simulink model "TwoLoopANNC_Integral_Paper"  (R2020b)
settings: Solver=ode4  StartTime=0.0  StopTime=100  FixedStep=1e-3  RelTol=1e-3
settings Model: Creator=Ivan Lopez  LastModifiedBy=Ivan Lopez

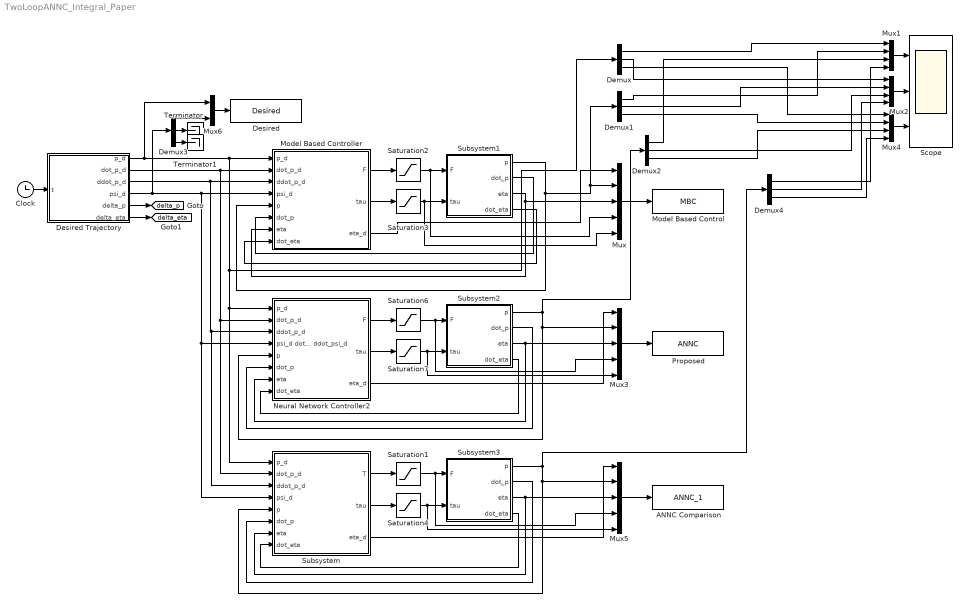
== system TwoLoopANNC_Integral_Paper ==
  ANNC Comparison : ToWorkspace  VariableName=ANNC_1  SaveFormat=Structure With Time  SampleTime=-1
  Clock : Clock
  Demux{,1..4} (5 alike) : Demux  Outputs=3
  Desired : ToWorkspace  VariableName=Desired  SaveFormat=Structure With Time  SampleTime=-1
  Desired Trajectory : MATLAB Function  TreatAsAtomicUnit=on
  Model Based Control : ToWorkspace  VariableName=MBC  SaveFormat=Structure With Time  SampleTime=-1
  Model Based Controller : Subsystem
  Mux : Mux  Inputs=5
  Mux1 : Mux
  Mux2 : Mux
  Mux3 : Mux  Inputs=5
  Mux4 : Mux
  Mux5 : Mux  Inputs=5
  Mux6 : Mux  Inputs=2
  Neural Network Controller2 : Subsystem
  Proposed : ToWorkspace  VariableName=ANNC  SaveFormat=Structure With Time  SampleTime=-1
  Saturation1 : Saturate  UpperLimit=34.4  LowerLimit=0
  Saturation2 : Saturate  UpperLimit=34.4  LowerLimit=0
  Saturation3 : Saturate  UpperLimit=1.72  LowerLimit=-1.72
  Saturation4 : Saturate  UpperLimit=1.72  LowerLimit=-1.72
  Saturation6 : Saturate  UpperLimit=34.4  LowerLimit=0
  Saturation7 : Saturate  UpperLimit=1.72  LowerLimit=-1.72
  Scope : Scope  NumInputPorts=3
  Subsystem : Subsystem
  Subsystem1 : Subsystem
  Subsystem2 : Subsystem
  Subsystem3 : Subsystem
  Terminator : Terminator
  Terminator1 : Terminator
  tag scope: delta_eta=global, delta_p=global
  wires:
  Neural Network Controller2/3(eta_d) -> Mux3/1
  Subsystem2/2(dot_p) -> Neural Network Controller2/6(dot_p)
  Subsystem2/4(dot_eta) -> Neural Network Controller2/8(dot_eta)
  Saturation3/1 -> Mux/5, Subsystem1/2(tau)
  Neural Network Controller2/2(tau) -> Saturation7/1
  Subsystem2/3(eta) -> Mux3/3, Neural Network Controller2/7(eta)
  Saturation7/1 -> Subsystem2/2(tau), Mux3/5
  Mux3/1 -> Proposed/1
  Subsystem1/1(p) -> Model Based Controller/5(p), Demux1/1, Mux/2
  Model Based Controller/3(eta_d) -> Mux/1
  Subsystem1/3(eta) -> Mux/3, Model Based Controller/7(eta)
  Model Based Controller/1(F) -> Saturation2/1
  Clock/1 -> Desired Trajectory/1(t)
  Saturation2/1 -> Mux/4, Subsystem1/1(F)
  Neural Network Controller2/1(F) -> Saturation6/1
  Desired Trajectory/3(ddot_p_d) -> Subsystem/3(ddot_p_d), Neural Network Controller2/3(ddot_p_d), Model Based Controller/3(ddot_p_d)
  Desired Trajectory/2(dot_p_d) -> Subsystem/2(dot_p_d), Neural Network Controller2/2(dot_p_d), Model Based Controller/2(dot_p_d)
  Mux/1 -> Model Based Control/1
  Saturation6/1 -> Subsystem2/1(F), Mux3/4
  Subsystem1/2(dot_p) -> Model Based Controller/6(dot_p)
  Desired Trajectory/1(p_d) -> Subsystem/1(p_d), Neural Network Controller2/1(p_d), Demux/1, Model Based Controller/1(p_d), Mux6/1
  Model Based Controller/2(tau) -> Saturation3/1
  Desired Trajectory/4(psi_d) -> Subsystem/4(psi_d), Neural Network Controller2/4(psi_d dot_psi_d ddot_psi_d), Model Based Controller/4(psi_d), Demux3/1
  Desired Trajectory/5(delta_p) -> [delta_p]
  Desired Trajectory/6(delta_eta) -> [delta_eta]
  Subsystem1/4(dot_eta) -> Model Based Controller/8(dot_eta)
  Mux1/1 -> Scope/1
  Mux2/1 -> Scope/2
  Mux4/1 -> Scope/3
  Demux/1 -> Mux1/1
  Demux1/1 -> Mux1/2
  Demux/2 -> Mux2/1
  Demux1/2 -> Mux2/2
  Demux/3 -> Mux4/1
  Demux1/3 -> Mux4/2
  Subsystem2/1(p) -> Demux2/1, Mux3/2, Neural Network Controller2/5(p)
  Demux2/1 -> Mux1/3
  Demux2/2 -> Mux2/3
  Demux2/3 -> Mux4/3
  Subsystem/3(eta_d) -> Mux5/1
  Subsystem3/1(p) -> Demux4/1, Subsystem/5(p), Mux5/2
  Saturation1/1 -> Subsystem3/1(F), Mux5/4
  Subsystem/1(T) -> Saturation1/1
  Subsystem3/4(dot_eta) -> Subsystem/8(dot_eta)
  Subsystem3/3(eta) -> Subsystem/7(eta), Mux5/3
  Mux5/1 -> ANNC Comparison/1
  Saturation4/1 -> Subsystem3/2(tau), Mux5/5
  Subsystem3/2(dot_p) -> Subsystem/6(dot_p)
  Subsystem/2(tau) -> Saturation4/1
  Mux6/1 -> Desired/1
  Demux3/1 -> Mux6/2
  Demux3/2 -> Terminator/1
  Demux3/3 -> Terminator1/1
  Demux4/1 -> Mux1/4
  Demux4/2 -> Mux2/4
  Demux4/3 -> Mux4/4

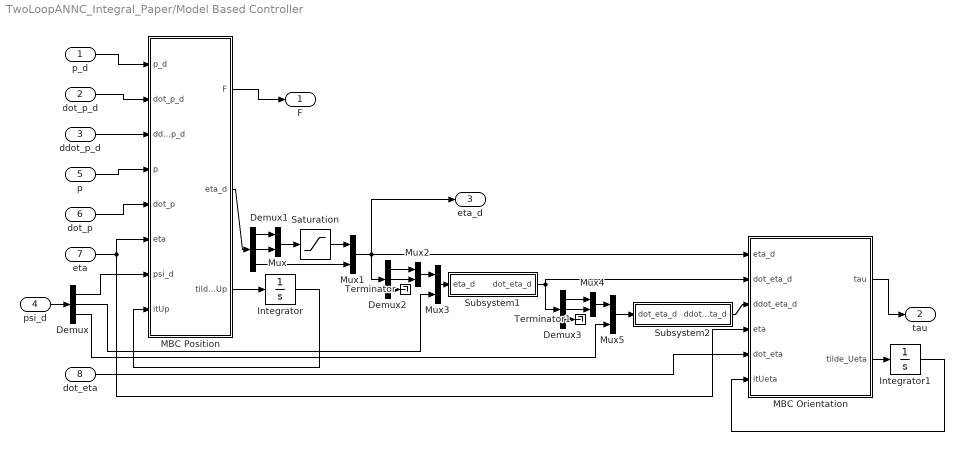
== system TwoLoopANNC_Integral_Paper/Model Based Controller ==
  p_d : Inport
  dot_p_d : Inport  Port=2
  ddot_p_d : Inport  Port=3
  psi_d : Inport  Port=4
  p : Inport  Port=5
  dot_p : Inport  Port=6
  eta : Inport  Port=7
  dot_eta : Inport  Port=8
  Demux{,1..3} (4 alike) : Demux  Outputs=3
  Integrator : Integrator  InitialCondition=[0;0;0]
  Integrator1 : Integrator  InitialCondition=[0;0;0]
  MBC Orientation : MATLAB Function  TreatAsAtomicUnit=on
  MBC Position : MATLAB Function  TreatAsAtomicUnit=on
  Mux{,1..5} (6 alike) : Mux  Inputs=2
  Saturation : Saturate  UpperLimit=20*pi/180  LowerLimit=-20*pi/180
  Subsystem1 : Subsystem
  Subsystem2 : Subsystem
  Terminator : Terminator
  Terminator1 : Terminator
  F : Outport
  tau : Outport  Port=2
  eta_d : Outport  Port=3
  wires:
  psi_d/1 -> Demux/1
  Subsystem1/1(dot_eta_d) -> Demux3/1, MBC Orientation/2(dot_eta_d)
  Subsystem2/1(ddot_eta_d) -> MBC Orientation/3(ddot_eta_d)
  MBC Position/1(F) -> F/1
  eta/1 -> MBC Orientation/4(eta), MBC Position/6(eta)
  ddot_p_d/1 -> MBC Position/3(ddot_p_d)
  MBC Orientation/1(tau) -> tau/1
  p/1 -> MBC Position/4(p)
  dot_p/1 -> MBC Position/5(dot_p)
  p_d/1 -> MBC Position/1(p_d)
  dot_eta/1 -> MBC Orientation/5(dot_eta)
  dot_p_d/1 -> MBC Position/2(dot_p_d)
  Mux1/1 -> Demux2/1, eta_d/1, MBC Orientation/1(eta_d)
  Demux/1 -> MBC Position/7(psi_d)
  MBC Position/2(eta_d) -> Demux1/1
  Demux1/2 -> Mux/2
  Demux1/1 -> Mux/1
  Mux/1 -> Saturation/1
  Saturation/1 -> Mux1/1
  Demux1/3 -> Mux1/2
  Demux2/2 -> Mux2/2
  Demux2/1 -> Mux2/1
  Mux2/1 -> Mux3/1
  Mux3/1 -> Subsystem1/1(eta_d)
  Demux/2 -> Mux3/2
  Demux2/3 -> Terminator/1
  Demux3/2 -> Mux4/2
  Mux5/1 -> Subsystem2/1(dot_eta_d)
  Mux4/1 -> Mux5/1
  Demux3/1 -> Mux4/1
  Demux3/3 -> Terminator1/1
  Demux/3 -> Mux5/2
  MBC Position/3(tilde_Up) -> Integrator/1
  Integrator/1 -> MBC Position/8(itUp)
  MBC Orientation/2(tilde_Ueta) -> Integrator1/1
  Integrator1/1 -> MBC Orientation/6(itUeta)

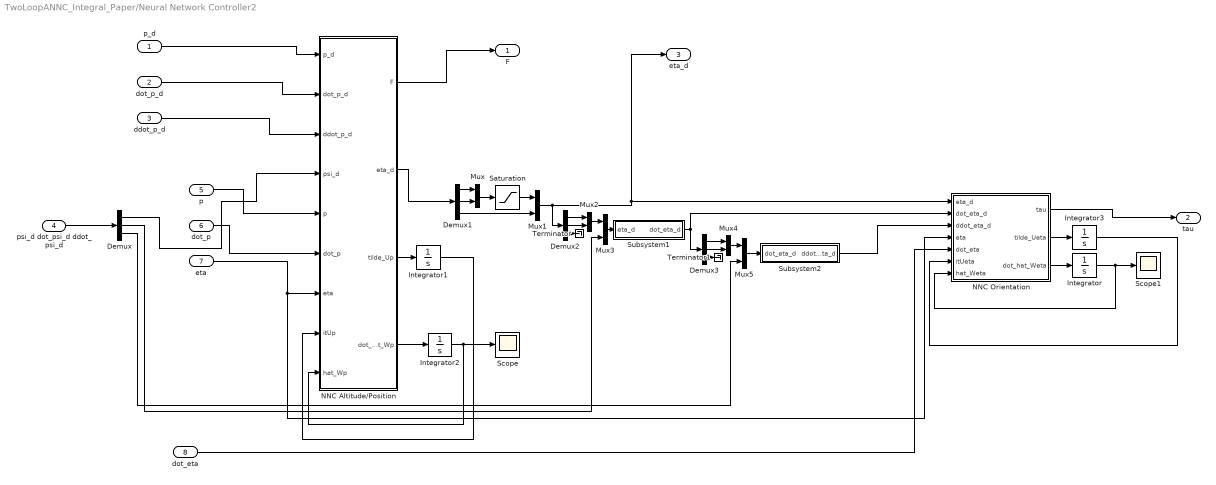
== system TwoLoopANNC_Integral_Paper/Neural Network Controller2 ==
  p_d : Inport
  dot_p_d : Inport  Port=2
  ddot_p_d : Inport  Port=3
  psi_d dot_psi_d ddot_psi_d : Inport  Port=4
  p : Inport  Port=5
  dot_p : Inport  Port=6
  eta : Inport  Port=7
  dot_eta : Inport  Port=8
  Demux{,1..3} (4 alike) : Demux  Outputs=3
  Integrator : Integrator  InitialCondition=zeros(10,3)
  Integrator1 : Integrator  InitialCondition=[0;0;0]
  Integrator2 : Integrator  InitialCondition=zeros(10,3)
  Integrator3 : Integrator  InitialCondition=[0;0;0]
  Mux{,1..5} (6 alike) : Mux  Inputs=2
  NNC Altitude/Position : MATLAB Function  TreatAsAtomicUnit=on
  NNC Orientation : MATLAB Function  TreatAsAtomicUnit=on
  Saturation : Saturate  UpperLimit=20*pi/180  LowerLimit=-20*pi/180
  Scope : Scope
  Scope1 : Scope
  Subsystem1 : Subsystem
  Subsystem2 : Subsystem
  Terminator : Terminator
  Terminator1 : Terminator
  F : Outport
  tau : Outport  Port=2
  eta_d : Outport  Port=3
  wires:
  NNC Altitude/Position/4(dot_hat_Wp) -> Integrator2/1
  Integrator/1 -> Scope1/1, NNC Orientation/7(hat_Weta)
  NNC Orientation/3(dot_hat_Weta) -> Integrator/1
  Integrator2/1 -> Scope/1, NNC Altitude/Position/9(hat_Wp)
  psi_d dot_psi_d ddot_psi_d/1 -> Demux/1
  Demux3/3 -> Terminator1/1
  Mux4/1 -> Mux5/1
  Demux3/1 -> Mux4/1
  Demux3/2 -> Mux4/2
  Demux/3 -> Mux5/2
  Demux/2 -> Mux3/2
  NNC Altitude/Position/2(eta_d) -> Demux1/1
  Demux1/1 -> Mux/1
  Demux2/2 -> Mux2/2
  Mux3/1 -> Subsystem1/1(eta_d)
  Demux1/3 -> Mux1/2
  Mux2/1 -> Mux3/1
  Demux2/3 -> Terminator/1
  Saturation/1 -> Mux1/1
  Demux1/2 -> Mux/2
  Mux5/1 -> Subsystem2/1(dot_eta_d)
  Demux2/1 -> Mux2/1
  Subsystem1/1(dot_eta_d) -> NNC Orientation/2(dot_eta_d), Demux3/1
  Mux1/1 -> NNC Orientation/1(eta_d), eta_d/1, Demux2/1
  Mux/1 -> Saturation/1
  Subsystem2/1(ddot_eta_d) -> NNC Orientation/3(ddot_eta_d)
  Demux/1 -> NNC Altitude/Position/4(psi_d)
  NNC Orientation/1(tau) -> tau/1
  NNC Altitude/Position/1(F) -> F/1
  dot_p_d/1 -> NNC Altitude/Position/2(dot_p_d)
  p_d/1 -> NNC Altitude/Position/1(p_d)
  eta/1 -> NNC Orientation/4(eta), NNC Altitude/Position/7(eta)
  p/1 -> NNC Altitude/Position/5(p)
  dot_p/1 -> NNC Altitude/Position/6(dot_p)
  dot_eta/1 -> NNC Orientation/5(dot_eta)
  ddot_p_d/1 -> NNC Altitude/Position/3(ddot_p_d)
  NNC Altitude/Position/3(tilde_Up) -> Integrator1/1
  Integrator1/1 -> NNC Altitude/Position/8(itUp)
  NNC Orientation/2(tilde_Ueta) -> Integrator3/1
  Integrator3/1 -> NNC Orientation/6(itUeta)

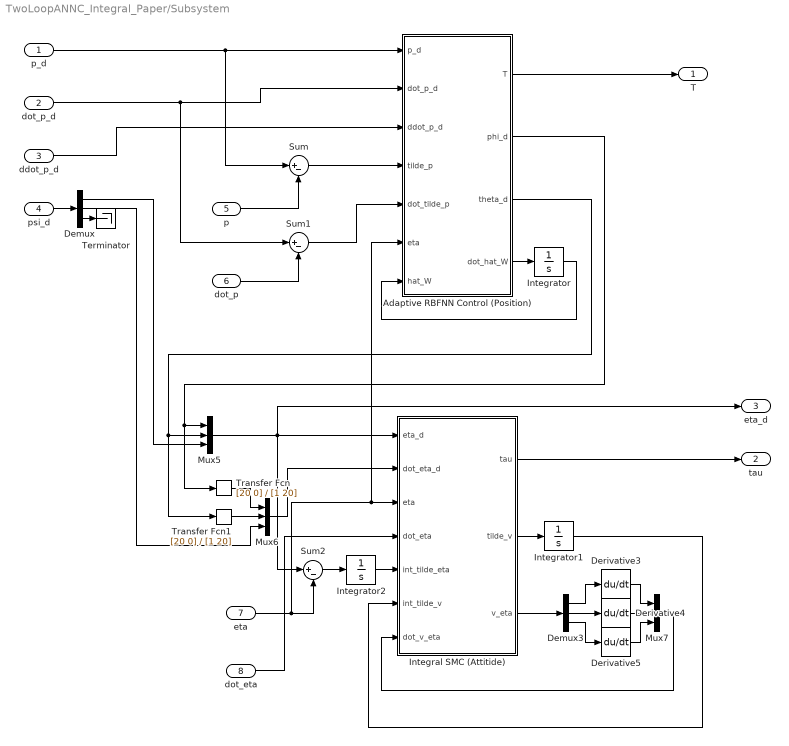
== system TwoLoopANNC_Integral_Paper/Subsystem ==
  p_d : Inport
  dot_p_d : Inport  Port=2
  ddot_p_d : Inport  Port=3
  psi_d : Inport  Port=4
  p : Inport  Port=5
  dot_p : Inport  Port=6
  eta : Inport  Port=7
  dot_eta : Inport  Port=8
  Adaptive RBFNN Control (Position) : MATLAB Function  TreatAsAtomicUnit=on
  Demux : Demux  Outputs=3
  Demux3 : Demux  Outputs=3
  Derivative3 : Derivative
  Derivative4 : Derivative
  Derivative5 : Derivative
  Integral SMC (Attitide) : MATLAB Function  TreatAsAtomicUnit=on
  Integrator : Integrator  InitialCondition=0.005*ones(7,3)
  Integrator1 : Integrator  InitialCondition=[0;0;0]
  Integrator2 : Integrator  InitialCondition=[0;0;0]
  Mux5 : Mux  Inputs=3
  Mux6 : Mux  Inputs=3
  Mux7 : Mux  Inputs=3
  Sum : Sum  Inputs=|+-
  Sum1 : Sum  Inputs=|+-
  Sum2 : Sum  Inputs=|+-
  Terminator : Terminator
  Transfer Fcn : TransferFcn  Numerator=[20 0]  Denominator=[1 20]
  Transfer Fcn1 : TransferFcn  Numerator=[20 0]  Denominator=[1 20]
  T : Outport
  tau : Outport  Port=2
  eta_d : Outport  Port=3
  wires:
  Demux3/1 -> Derivative3/1
  Adaptive RBFNN Control (Position)/3(theta_d) -> Transfer Fcn1/1, Mux5/2
  Integral SMC (Attitide)/1(tau) -> tau/1
  Demux/1 -> Mux5/3
  Adaptive RBFNN Control (Position)/2(phi_d) -> Transfer Fcn/1, Mux5/1
  eta/1 -> Adaptive RBFNN Control (Position)/6(eta), Integral SMC (Attitide)/3(eta), Sum2/2
  Mux7/1 -> Integral SMC (Attitide)/7(dot_v_eta)
  Demux3/3 -> Derivative5/1
  Sum1/1 -> Adaptive RBFNN Control (Position)/5(dot_tilde_p)
  Integral SMC (Attitide)/2(tilde_v) -> Integrator1/1
  Integrator1/1 -> Integral SMC (Attitide)/6(int_tilde_v)
  Derivative5/1 -> Mux7/3
  Mux5/1 -> eta_d/1, Sum2/1, Integral SMC (Attitide)/1(eta_d)
  Adaptive RBFNN Control (Position)/4(dot_hat_W) -> Integrator/1
  Transfer Fcn/1 -> Mux6/1
  Integral SMC (Attitide)/3(v_eta) -> Demux3/1
  Demux3/2 -> Derivative4/1
  dot_p_d/1 -> Sum1/1, Adaptive RBFNN Control (Position)/2(dot_p_d)
  Sum2/1 -> Integrator2/1
  Integrator/1 -> Adaptive RBFNN Control (Position)/7(hat_W)
  Derivative3/1 -> Mux7/1
  Derivative4/1 -> Mux7/2
  p/1 -> Sum/2
  dot_eta/1 -> Integral SMC (Attitide)/4(dot_eta)
  Transfer Fcn1/1 -> Mux6/2
  dot_p/1 -> Sum1/2
  Sum/1 -> Adaptive RBFNN Control (Position)/4(tilde_p)
  Mux6/1 -> Integral SMC (Attitide)/2(dot_eta_d)
  Integrator2/1 -> Integral SMC (Attitide)/5(int_tilde_eta)
  p_d/1 -> Sum/1, Adaptive RBFNN Control (Position)/1(p_d)
  ddot_p_d/1 -> Adaptive RBFNN Control (Position)/3(ddot_p_d)
  Adaptive RBFNN Control (Position)/1(T) -> T/1
  psi_d/1 -> Demux/1
  Demux/2 -> Mux6/3
  Demux/3 -> Terminator/1

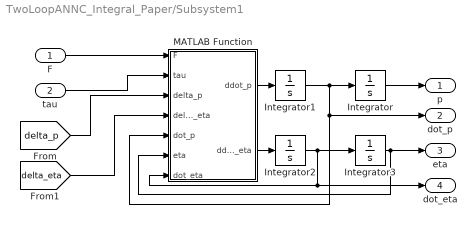
== system TwoLoopANNC_Integral_Paper/Subsystem1 ==
  F : Inport
  tau : Inport  Port=2
  Integrator : Integrator  InitialCondition=[0;0;0.3]  LimitOutput=on  UpperSaturationLimit=[inf;inf;inf]  LowerSaturationLimit=[-inf;-inf;0.3]
  Integrator1 : Integrator  InitialCondition=[0;0;0]
  Integrator2 : Integrator  InitialCondition=[0;0;0]
  Integrator3 : Integrator  InitialCondition=[0;0;0]  LimitOutput=on  UpperSaturationLimit=[pi/2; pi/2; inf]  LowerSaturationLimit=[-pi/2; -pi/2; -inf]
  MATLAB Function : MATLAB Function  TreatAsAtomicUnit=on
  p : Outport
  dot_p : Outport  Port=2
  eta : Outport  Port=3
  dot_eta : Outport  Port=4
  wires:
  [delta_p] -> MATLAB Function/3(delta_p)
  [delta_eta] -> MATLAB Function/4(delta_eta)
  F/1 -> MATLAB Function/1(F)
  Integrator3/1 -> MATLAB Function/6(eta), eta/1
  Integrator1/1 -> dot_p/1, MATLAB Function/5(dot_p), Integrator/1
  MATLAB Function/2(ddot_eta) -> Integrator2/1
  MATLAB Function/1(ddot_p) -> Integrator1/1
  tau/1 -> MATLAB Function/2(tau)
  Integrator2/1 -> Integrator3/1, dot_eta/1, MATLAB Function/7(dot_eta)
  Integrator/1 -> p/1

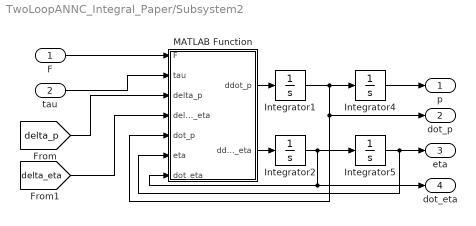
== system TwoLoopANNC_Integral_Paper/Subsystem2 ==
  F : Inport
  tau : Inport  Port=2
  Integrator1 : Integrator  InitialCondition=[0;0;0]
  Integrator2 : Integrator  InitialCondition=[0;0;0]
  Integrator4 : Integrator  InitialCondition=[0;0;0.3]  LimitOutput=on  UpperSaturationLimit=[inf;inf;inf]  LowerSaturationLimit=[-inf;-inf;0.3]
  Integrator5 : Integrator  InitialCondition=[0;0;0]  LimitOutput=on  UpperSaturationLimit=[pi/2; pi/2; inf]  LowerSaturationLimit=[-pi/2; -pi/2; -inf]
  MATLAB Function : MATLAB Function  TreatAsAtomicUnit=on
  p : Outport
  dot_p : Outport  Port=2
  eta : Outport  Port=3
  dot_eta : Outport  Port=4
  wires:
  [delta_p] -> MATLAB Function/3(delta_p)
  [delta_eta] -> MATLAB Function/4(delta_eta)
  F/1 -> MATLAB Function/1(F)
  MATLAB Function/2(ddot_eta) -> Integrator2/1
  MATLAB Function/1(ddot_p) -> Integrator1/1
  tau/1 -> MATLAB Function/2(tau)
  Integrator4/1 -> p/1
  Integrator5/1 -> eta/1, MATLAB Function/6(eta)
  Integrator1/1 -> Integrator4/1, dot_p/1, MATLAB Function/5(dot_p)
  Integrator2/1 -> Integrator5/1, dot_eta/1, MATLAB Function/7(dot_eta)

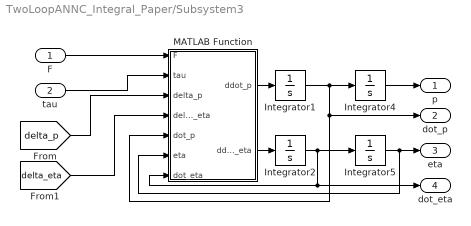
== system TwoLoopANNC_Integral_Paper/Subsystem3 ==
  F : Inport
  tau : Inport  Port=2
  Integrator1 : Integrator  InitialCondition=[0;0;0]
  Integrator2 : Integrator  InitialCondition=[0;0;0]
  Integrator4 : Integrator  InitialCondition=[0;0;0.3]  LimitOutput=on  UpperSaturationLimit=[inf;inf;inf]  LowerSaturationLimit=[-inf;-inf;0.3]
  Integrator5 : Integrator  InitialCondition=[0;0;0]  LimitOutput=on  UpperSaturationLimit=[pi/2; pi/2; inf]  LowerSaturationLimit=[-pi/2; -pi/2; -inf]
  MATLAB Function : MATLAB Function  TreatAsAtomicUnit=on
  p : Outport
  dot_p : Outport  Port=2
  eta : Outport  Port=3
  dot_eta : Outport  Port=4
  wires:
  [delta_p] -> MATLAB Function/3(delta_p)
  [delta_eta] -> MATLAB Function/4(delta_eta)
  F/1 -> MATLAB Function/1(F)
  MATLAB Function/2(ddot_eta) -> Integrator2/1
  MATLAB Function/1(ddot_p) -> Integrator1/1
  tau/1 -> MATLAB Function/2(tau)
  Integrator4/1 -> p/1
  Integrator5/1 -> eta/1, MATLAB Function/6(eta)
  Integrator1/1 -> Integrator4/1, dot_p/1, MATLAB Function/5(dot_p)
  Integrator2/1 -> Integrator5/1, dot_eta/1, MATLAB Function/7(dot_eta)

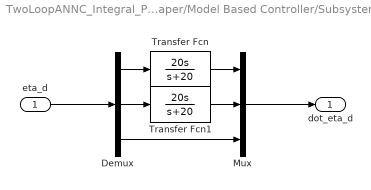
== system TwoLoopANNC_Integral_Paper/Model Based Controller/Subsystem1 ==
  eta_d : Inport
  Demux : Demux  Outputs=3
  Mux : Mux  Inputs=3
  Transfer Fcn : TransferFcn  Numerator=[20 0]  Denominator=[1 20]
  Transfer Fcn1 : TransferFcn  Numerator=[20 0]  Denominator=[1 20]
  dot_eta_d : Outport
  wires:
  Demux/2 -> Transfer Fcn1/1
  Demux/3 -> Mux/3
  Demux/1 -> Transfer Fcn/1
  Transfer Fcn/1 -> Mux/1
  Transfer Fcn1/1 -> Mux/2
  Mux/1 -> dot_eta_d/1
  eta_d/1 -> Demux/1

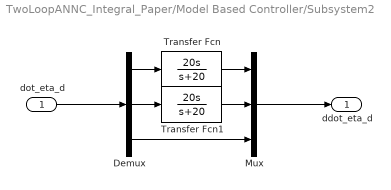
== system TwoLoopANNC_Integral_Paper/Model Based Controller/Subsystem2 ==
  dot_eta_d : Inport
  Demux : Demux  Outputs=3
  Mux : Mux  Inputs=3
  Transfer Fcn : TransferFcn  Numerator=[20 0]  Denominator=[1 20]
  Transfer Fcn1 : TransferFcn  Numerator=[20 0]  Denominator=[1 20]
  ddot_eta_d : Outport
  wires:
  Demux/3 -> Mux/3
  Transfer Fcn1/1 -> Mux/2
  Demux/2 -> Transfer Fcn1/1
  Demux/1 -> Transfer Fcn/1
  Transfer Fcn/1 -> Mux/1
  dot_eta_d/1 -> Demux/1
  Mux/1 -> ddot_eta_d/1

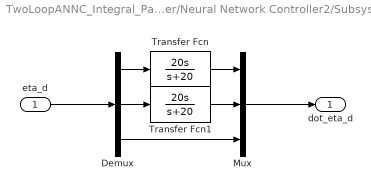
== system TwoLoopANNC_Integral_Paper/Neural Network Controller2/Subsystem1 ==
  eta_d : Inport
  Demux : Demux  Outputs=3
  Mux : Mux  Inputs=3
  Transfer Fcn : TransferFcn  Numerator=[20 0]  Denominator=[1 20]
  Transfer Fcn1 : TransferFcn  Numerator=[20 0]  Denominator=[1 20]
  dot_eta_d : Outport
  wires:
  Demux/2 -> Transfer Fcn1/1
  Demux/3 -> Mux/3
  Demux/1 -> Transfer Fcn/1
  Transfer Fcn/1 -> Mux/1
  Transfer Fcn1/1 -> Mux/2
  Mux/1 -> dot_eta_d/1
  eta_d/1 -> Demux/1

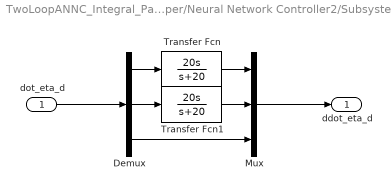
== system TwoLoopANNC_Integral_Paper/Neural Network Controller2/Subsystem2 ==
  dot_eta_d : Inport
  Demux : Demux  Outputs=3
  Mux : Mux  Inputs=3
  Transfer Fcn : TransferFcn  Numerator=[20 0]  Denominator=[1 20]
  Transfer Fcn1 : TransferFcn  Numerator=[20 0]  Denominator=[1 20]
  ddot_eta_d : Outport
  wires:
  Demux/3 -> Mux/3
  Transfer Fcn1/1 -> Mux/2
  Demux/2 -> Transfer Fcn1/1
  Demux/1 -> Transfer Fcn/1
  Transfer Fcn/1 -> Mux/1
  dot_eta_d/1 -> Demux/1
  Mux/1 -> ddot_eta_d/1

== matlab function TwoLoopANNC_Integral_Paper/Subsystem3/MATLAB Function ==
  data: F input; ddot_p output; ddot_eta output; tau input; delta_p input; delta_eta input; dot_p input; eta input; dot_eta input
function [ddot_p, ddot_eta] = fcn(F, tau, delta_p, delta_eta, dot_p, eta, dot_eta)

m  = 1.79;
g  = 9.81;
Ixx = 0.03; Iyy = 0.03; Izz = 0.04;
dx = 0.002; dy = 0.002; dz = 0.004;
d_phi = 0.002; d_theta = 0.002; d_psi = 0.004;
I  = diag([Ixx Iyy Izz]);
Dp = diag([dx dy dz]);
Dn = diag([d_phi d_theta d_psi]);
Vz = [0; 0; 1];

phi     = eta(1);     theta     = eta(2);     psi = eta(3);
dot_phi = dot_eta(1); dot_theta = dot_eta(2);

R = [cos(theta)*cos(psi)  sin(phi)*sin(theta)*cos(psi)-cos(phi)*sin(psi)  cos(phi)*sin(theta)*cos(psi)+sin(phi)*sin(psi)
     cos(theta)*sin(psi)  sin(phi)*sin(theta)*sin(psi)+cos(phi)*cos(psi)  cos(phi)*sin(theta)*sin(psi)-sin(phi)*cos(psi)
     -sin(theta)          sin(phi)*cos(theta)                             cos(phi)*cos(theta)];
 
% W = [1  sin(phi)*tan(theta)  cos(phi)*tan(theta)
%      0  cos(phi)             -sin(phi)
%      0  sin(phi)/cos(theta)  cos(phi)/cos(theta)];

iW = [1 0         -sin(theta)
      0 cos(phi)  cos(theta)*sin(phi)
      0 -sin(phi) cos(theta)*cos(phi)];
 
dot_W = [0  (cos(phi)*tan(theta))+((sin(phi)*dot_theta)/(cos(theta)^2))                     ((cos(phi)*dot_theta)/(cos(theta)^2))-(sin(phi)*tan(theta)*dot_phi)
         0  -sin(phi)*dot_phi                                                               -cos(phi)*dot_phi
         0  ((cos(phi)*cos(theta)*dot_phi)+(sin(phi)*sin(theta)*dot_theta))/(cos(theta)^2)  ((cos(phi)*sin(theta)*dot_theta)-(sin(phi)*cos(theta)*dot_phi))/(cos(theta)^2)];
  
iWdot_eta = iW*dot_eta;

SiWdot_eta = [0              -iWdot_eta(3)  iWdot_eta(2)
              iWdot_eta(3)   0              -iWdot_eta(1)
              -iWdot_eta(2)  iWdot_eta(1)   0];

M = iW'*I*iW;
C = iW'*(SiWdot_eta*I - I*iW*dot_W)*iW;

ddot_p   = (R*Vz*F + delta_p - m*g*Vz - Dp*dot_p)/m;
ddot_eta = M\(iW'*tau + delta_eta - C*dot_eta - Dn*dot_eta);

== matlab function TwoLoopANNC_Integral_Paper/Neural Network Controller2/NNC Altitude//Position ==
  data: p_d input; F output; dot_p_d input; ddot_p_d input; psi_d input; p input; dot_p input; eta input; itUp input; eta_d output; tilde_Up output; dot_hat_Wp output; hat_Wp input
function [F, eta_d, tilde_Up, dot_hat_Wp] = fcn(p_d, dot_p_d, ddot_p_d, psi_d, p, dot_p, eta, itUp, hat_Wp)
m       = 1.79;
g       = 9.81;
gz      = [0; 0; g];
phi     = eta(1);
theta   = eta(2);
e_p     = p_d - p;
dot_e_p = dot_p_d - dot_p;
%% Position controller %%%
%%% Gains %%%
hat_m = 0.85*m; % mass uncertainty
KUp   = diag([0.75 0.75 10]);
Kip   = diag([0.2 0.2 0.75]);
Kp    = diag([1.75 1.75 12]);

Up       = dot_p_d + Kp*e_p;
dot_Up   = ddot_p_d + Kp*dot_e_p;
tilde_Up = Up - dot_p;
%%% Neural Network Structure %%%
gamma_p   = [1; dot_p; eta; dot_Up];
neurons_p = 10;
V_p = [0.6294   -0.0292    0.4863   -0.9311    0.3102    0.9186    0.2321   -0.8921   -0.6687    0.9923
    0.8116    0.6006   -0.2155   -0.1225   -0.6748    0.0944   -0.0534    0.0616    0.2040   -0.8436
   -0.7460   -0.7162    0.3110   -0.2369   -0.7620   -0.7228   -0.2967    0.5583   -0.4741   -0.1146
    0.8268   -0.1565   -0.6576    0.5310   -0.0033   -0.7014    0.6617    0.8680    0.3082   -0.7867
    0.2647    0.8315    0.4121    0.5904    0.9195   -0.4850    0.1705   -0.7402    0.3784    0.9238
   -0.8049    0.5844   -0.9363   -0.6263   -0.3192    0.6814    0.0994    0.1376    0.4963   -0.9907
   -0.4430    0.9190   -0.4462   -0.0205    0.1705   -0.4914    0.8344   -0.0612   -0.0989    0.5498
    0.0938    0.3115   -0.9077   -0.1088   -0.5524    0.6286   -0.4283   -0.9762   -0.8324    0.6346
    0.9150   -0.9286   -0.8057    0.2926    0.5025   -0.5130    0.5144   -0.3258   -0.5420    0.7374
    0.9298    0.6983    0.6469    0.4187   -0.4898    0.8585    0.5075   -0.6756    0.8267   -0.8311];
sigma_p = tanh(V_p'*gamma_p);
%%% Neural Network Gains %%%
flag_NN = 1; % <------------ On/Off NN
N_p     = 0.8*eye(neurons_p);   % 2   % 3.5 % 2.2  % 2.2 % 2.2  % 0.65
kp      = 0.001;                 % 0.1 % 0.4 % 1.25 % 1.2 % 1.15 % 0.001
a_p     = 0.001*diag([1 1 1]);
%%% Controller %%%
F_p        = KUp*tilde_Up + Kip*itUp + hat_m*(dot_Up + gz) + flag_NN*(hat_Wp'*sigma_p + a_p*sign(tilde_Up));
dot_hat_Wp = N_p*(sigma_p*tilde_Up' - kp*norm(tilde_Up)*hat_Wp);
theta_d    = atan((F_p(1)*cos(psi_d) + F_p(2)*sin(psi_d))/F_p(3));
phi_d      = atan(cos(theta_d)*(F_p(1)*sin(psi_d) - F_p(2)*cos(psi_d))/F_p(3));
F          = F_p(3)/(cos(phi)*cos(theta));
eta_d      = [phi_d; theta_d; psi_d];

== matlab function TwoLoopANNC_Integral_Paper/Neural Network Controller2/NNC Orientation ==
  settings: updateMethod=DISCRETE
  data: eta_d input; tau output; tilde_Ueta output; dot_eta_d input; ddot_eta_d input; eta input; dot_eta input; itUeta input; hat_Weta input; dot_hat_Weta output
function [tau, tilde_Ueta, dot_hat_Weta] = fcn(eta_d, dot_eta_d, ddot_eta_d, eta, dot_eta, itUeta, hat_Weta)

phi = eta(1) ; theta = eta(2);
%% Gains
K_Ueta = 2*diag([1 1 1]);
K_ieta = 0.05*diag([1 1 1]);
K_eta  = 5*diag([1 1 1]);
%% Attitude Controller
e_eta     = eta_d - eta;
dot_e_eta = dot_eta_d - dot_eta;

Ueta       = dot_eta_d + K_eta*e_eta;
dot_Ueta   = ddot_eta_d + K_eta*dot_e_eta;
tilde_Ueta = Ueta - dot_eta;

gamma_eta = [1; eta; dot_eta; dot_Ueta];
neurons_eta = 10;
V_eta = [0.6294   -0.0292    0.4863   -0.9311    0.3102    0.9186    0.2321   -0.8921   -0.6687    0.9923
    0.8116    0.6006   -0.2155   -0.1225   -0.6748    0.0944   -0.0534    0.0616    0.2040   -0.8436
   -0.7460   -0.7162    0.3110   -0.2369   -0.7620   -0.7228   -0.2967    0.5583   -0.4741   -0.1146
    0.8268   -0.1565   -0.6576    0.5310   -0.0033   -0.7014    0.6617    0.8680    0.3082   -0.7867
    0.2647    0.8315    0.4121    0.5904    0.9195   -0.4850    0.1705   -0.7402    0.3784    0.9238
   -0.8049    0.5844   -0.9363   -0.6263   -0.3192    0.6814    0.0994    0.1376    0.4963   -0.9907
   -0.4430    0.9190   -0.4462   -0.0205    0.1705   -0.4914    0.8344   -0.0612   -0.0989    0.5498
    0.0938    0.3115   -0.9077   -0.1088   -0.5524    0.6286   -0.4283   -0.9762   -0.8324    0.6346
    0.9150   -0.9286   -0.8057    0.2926    0.5025   -0.5130    0.5144   -0.3258   -0.5420    0.7374
    0.9298    0.6983    0.6469    0.4187   -0.4898    0.8585    0.5075   -0.6756    0.8267   -0.8311];

sigma_eta = tanh(V_eta'*gamma_eta);
N_eta = 1.85*eye(neurons_eta);% 22  % 22   % 12   % 30
keta  = 0.003;                % 3.9 % 3.95 % 3.95 % 3.95
a_eta = 0.001*diag([1 1 1]);

W = [1  sin(phi)*tan(theta)  cos(phi)*tan(theta)
     0  cos(phi)             -sin(phi)
     0  sin(phi)/cos(theta)  cos(phi)/cos(theta)];

tau_eta = K_Ueta*tilde_Ueta + K_ieta*itUeta + hat_Weta'*sigma_eta + a_eta*sign(tilde_Ueta);
tau     = W'*tau_eta;
dot_hat_Weta = N_eta*(sigma_eta*tilde_Ueta' - keta*norm(tilde_Ueta)*hat_Weta);

== matlab function TwoLoopANNC_Integral_Paper/Subsystem2/MATLAB Function ==
  data: F input; ddot_p output; ddot_eta output; tau input; delta_p input; delta_eta input; dot_p input; eta input; dot_eta input
function [ddot_p, ddot_eta] = fcn(F, tau, delta_p, delta_eta, dot_p, eta, dot_eta)

m  = 1.79;
g  = 9.81;
Ixx = 0.03; Iyy = 0.03; Izz = 0.04;
dx = 0.002; dy = 0.002; dz = 0.004;
d_phi = 0.002; d_theta = 0.002; d_psi = 0.004;
I  = diag([Ixx Iyy Izz]);
Dp = diag([dx dy dz]);
Dn = diag([d_phi d_theta d_psi]);
Vz = [0; 0; 1];

phi     = eta(1);     theta     = eta(2);     psi = eta(3);
dot_phi = dot_eta(1); dot_theta = dot_eta(2);

R = [cos(theta)*cos(psi)  sin(phi)*sin(theta)*cos(psi)-cos(phi)*sin(psi)  cos(phi)*sin(theta)*cos(psi)+sin(phi)*sin(psi)
     cos(theta)*sin(psi)  sin(phi)*sin(theta)*sin(psi)+cos(phi)*cos(psi)  cos(phi)*sin(theta)*sin(psi)-sin(phi)*cos(psi)
     -sin(theta)          sin(phi)*cos(theta)                             cos(phi)*cos(theta)];
 
% W = [1  sin(phi)*tan(theta)  cos(phi)*tan(theta)
%      0  cos(phi)             -sin(phi)
%      0  sin(phi)/cos(theta)  cos(phi)/cos(theta)];

iW = [1 0         -sin(theta)
      0 cos(phi)  cos(theta)*sin(phi)
      0 -sin(phi) cos(theta)*cos(phi)];
 
dot_W = [0  (cos(phi)*tan(theta))+((sin(phi)*dot_theta)/(cos(theta)^2))                     ((cos(phi)*dot_theta)/(cos(theta)^2))-(sin(phi)*tan(theta)*dot_phi)
         0  -sin(phi)*dot_phi                                                               -cos(phi)*dot_phi
         0  ((cos(phi)*cos(theta)*dot_phi)+(sin(phi)*sin(theta)*dot_theta))/(cos(theta)^2)  ((cos(phi)*sin(theta)*dot_theta)-(sin(phi)*cos(theta)*dot_phi))/(cos(theta)^2)];
  
iWdot_eta = iW*dot_eta;

SiWdot_eta = [0              -iWdot_eta(3)  iWdot_eta(2)
              iWdot_eta(3)   0              -iWdot_eta(1)
              -iWdot_eta(2)  iWdot_eta(1)   0];

M = iW'*I*iW;
C = iW'*(SiWdot_eta*I - I*iW*dot_W)*iW;

ddot_p   = (R*Vz*F + delta_p - m*g*Vz - Dp*dot_p)/m;
ddot_eta = M\(iW'*tau + delta_eta - C*dot_eta - Dn*dot_eta);

== matlab function TwoLoopANNC_Integral_Paper/Model Based Controller/MBC Orientation ==
  data: eta_d input; tau output; dot_eta_d input; ddot_eta_d input; eta input; dot_eta input; itUeta input; tilde_Ueta output
function [tau, tilde_Ueta] = fcn(eta_d, dot_eta_d, ddot_eta_d, eta, dot_eta,itUeta)

phi     = eta(1);     theta = eta(2);
dot_phi = dot_eta(1); dot_theta = dot_eta(2);
Ixx = 0.03; Iyy = 0.03; Izz = 0.04;
d_phi = 0.002; d_theta = 0.002; d_psi = 0.004;
I  = diag([Ixx Iyy Izz]);
Dn = diag([d_phi d_theta d_psi]);
%% Gains
K1eta = 2*diag([1 1 1]);
K2eta = 0.05*diag([1 1 1]);
K3eta = 5*diag([1 1 1]);

e_eta     = eta_d - eta;
dot_e_eta = dot_eta_d - dot_eta;

Ueta     = dot_eta_d + K3eta*e_eta;
dot_Ueta = ddot_eta_d + K3eta*dot_e_eta;

tilde_Ueta = Ueta - dot_eta;

W = [1  sin(phi)*tan(theta)  cos(phi)*tan(theta)
     0  cos(phi)             -sin(phi)
     0  sin(phi)/cos(theta)  cos(phi)/cos(theta)];

iW = [1 0         -sin(theta)
      0 cos(phi)  cos(theta)*sin(phi)
      0 -sin(phi) cos(theta)*cos(phi)];
 
dot_W = [0  (cos(phi)*tan(theta))+((sin(phi)*dot_theta)/(cos(theta)^2))                     ((cos(phi)*dot_theta)/(cos(theta)^2))-(sin(phi)*tan(theta)*dot_phi)
         0  -sin(phi)*dot_phi                                                               -cos(phi)*dot_phi
         0  ((cos(phi)*cos(theta)*dot_phi)+(sin(phi)*sin(theta)*dot_theta))/(cos(theta)^2)  ((cos(phi)*sin(theta)*dot_theta)-(sin(phi)*cos(theta)*dot_phi))/(cos(theta)^2)];
  
iWdot_eta = iW*dot_eta;

SiWdot_eta = [0              -iWdot_eta(3)  iWdot_eta(2)
              iWdot_eta(3)   0              -iWdot_eta(1)
              -iWdot_eta(2)  iWdot_eta(1)   0];

M = iW'*I*iW;
C = iW'*(SiWdot_eta*I - I*iW*dot_W)*iW;
tau = W'*(K1eta*tilde_Ueta + K2eta*itUeta + (C + Dn)*dot_eta + M*dot_Ueta);

== matlab function TwoLoopANNC_Integral_Paper/Subsystem1/MATLAB Function ==
  data: F input; ddot_p output; ddot_eta output; tau input; delta_p input; delta_eta input; dot_p input; eta input; dot_eta input
function [ddot_p, ddot_eta] = fcn(F, tau, delta_p, delta_eta, dot_p, eta, dot_eta)

m  = 1.79;
g  = 9.81;
Ixx = 0.03; Iyy = 0.03; Izz = 0.04;
dx = 0.002; dy = 0.002; dz = 0.004;
d_phi = 0.002; d_theta = 0.002; d_psi = 0.004;
I  = diag([Ixx Iyy Izz]);
Dp = diag([dx dy dz]);
Dn = diag([d_phi d_theta d_psi]);
Vz = [0; 0; 1];

phi     = eta(1);     theta     = eta(2);     psi = eta(3);
dot_phi = dot_eta(1); dot_theta = dot_eta(2);

R = [cos(theta)*cos(psi)  sin(phi)*sin(theta)*cos(psi)-cos(phi)*sin(psi)  cos(phi)*sin(theta)*cos(psi)+sin(phi)*sin(psi)
     cos(theta)*sin(psi)  sin(phi)*sin(theta)*sin(psi)+cos(phi)*cos(psi)  cos(phi)*sin(theta)*sin(psi)-sin(phi)*cos(psi)
     -sin(theta)          sin(phi)*cos(theta)                             cos(phi)*cos(theta)];
 
% W = [1  sin(phi)*tan(theta)  cos(phi)*tan(theta)
%      0  cos(phi)             -sin(phi)
%      0  sin(phi)/cos(theta)  cos(phi)/cos(theta)];

iW = [1 0         -sin(theta)
      0 cos(phi)  cos(theta)*sin(phi)
      0 -sin(phi) cos(theta)*cos(phi)];
 
dot_W = [0  (cos(phi)*tan(theta))+((sin(phi)*dot_theta)/(cos(theta)^2))                     ((cos(phi)*dot_theta)/(cos(theta)^2))-(sin(phi)*tan(theta)*dot_phi)
         0  -sin(phi)*dot_phi                                                               -cos(phi)*dot_phi
         0  ((cos(phi)*cos(theta)*dot_phi)+(sin(phi)*sin(theta)*dot_theta))/(cos(theta)^2)  ((cos(phi)*sin(theta)*dot_theta)-(sin(phi)*cos(theta)*dot_phi))/(cos(theta)^2)];
  
iWdot_eta = iW*dot_eta;

SiWdot_eta = [0              -iWdot_eta(3)  iWdot_eta(2)
              iWdot_eta(3)   0              -iWdot_eta(1)
              -iWdot_eta(2)  iWdot_eta(1)   0];

M = iW'*I*iW;
C = iW'*(SiWdot_eta*I - I*iW*dot_W)*iW;

ddot_p   = (R*Vz*F + delta_p - m*g*Vz - Dp*dot_p)/m;
ddot_eta = M\(iW'*tau + delta_eta - C*dot_eta - Dn*dot_eta);

== matlab function TwoLoopANNC_Integral_Paper/Model Based Controller/MBC Position ==
  data: p_d input; F output; dot_p_d input; ddot_p_d input; p input; dot_p input; eta input; psi_d input; eta_d output; itUp input; tilde_Up output
function [F, eta_d, tilde_Up] = fcn(p_d, dot_p_d, ddot_p_d, p, dot_p, eta, psi_d, itUp)
m  = 0.85*1.79;
g  = 9.81;
gz = [0; 0; g];
dx = 0.002; dy = 0.002; dz = 0.004;
Dp = diag([dx dy dz]);
phi = eta(1) ; theta = eta(2);

e_p     = p_d - p;
dot_e_p = dot_p_d - dot_p;
%% Position Controller
%Gains
K1p = diag([0.75 0.75 10]);
K2p = diag([0.2 0.2 0.75]);
K3p = diag([1.75 1.75 12]);

Up       = dot_p_d + K3p*e_p;
dot_Up   = ddot_p_d + K3p*dot_e_p;
tilde_Up = Up - dot_p;

F_p     = K1p*tilde_Up + K2p*itUp + m*(dot_Up + gz) + Dp*dot_p + K1p*tilde_Up;
theta_d = atan((F_p(1)*cos(psi_d) + F_p(2)*sin(psi_d))/F_p(3));
phi_d   = atan(cos(theta_d)*(F_p(1)*sin(psi_d) - F_p(2)*cos(psi_d))/F_p(3));
F       = F_p(3)/(cos(phi)*cos(theta));

eta_d = [phi_d; theta_d; psi_d];

== matlab function TwoLoopANNC_Integral_Paper/Desired Trajectory ==
  data: t input; p_d output; dot_p_d output; ddot_p_d output; psi_d output; delta_p output; delta_eta output
function [p_d, dot_p_d, ddot_p_d, psi_d, delta_p, delta_eta] = fcn(t)
z0    = 0.3;
h     = 1.4;
%% Circunferencia
% ampx = 1;
% ampy = 1;
% ampz = 0.1;
% amps = 10*pi/180;
% frecx = 2*pi/5;
% frecy = 2*pi/5;
% frecz = 2*pi/5;
% frecs = 2*pi/5;

%% Lemniscata 1
% 
% ampx = 0.5;
% ampy = 1;
% ampz = 0.4;
% amps = 5*pi/180;
% frecx = 2*pi/4;
% frecy = 2*pi/8;
% frecz = 2*pi/4;
% frecs = 2*pi/4;
% 
% x_d      = ampx*sin(frecx*t);
% dot_x_d  = ampx*frecx*cos(frecx*t);
% ddot_x_d = -ampx*frecx^2*sin(frecx*t);
% 
% y_d      = ampy*cos(frecy*t);
% dot_y_d  = -ampy*frecy*sin(frecy*t);
% ddot_y_d = -ampy*frecy^2*cos(frecy*t);
% 
% if (t>=0 && t<=5)
%     z_d      = h - (h - z0)*exp(-ampz*t^3);
%     dot_z_d  = 3*ampz*t^2*(h - z0)*exp(-ampz*t^3);
%     ddot_z_d = (3*ampz*t^3 - 2)*3*ampz*t*(z0 - h)*exp(-ampz*t^3);
% else
%     z_d      = (h - ampz) + ampz*sin(frecz*t);
%     dot_z_d  = ampz*frecz*cos(frecz*t);
%     ddot_z_d = -ampz*frecz^2*sin(frecz*t);
% end
% 
% psi_d      = [amps*sin(frecs*t)
%               amps*frecs*cos(frecs*t)
%              -amps*frecs^2*sin(frecs*t)];
%        
% p_d      = [x_d; y_d; z_d];
% dot_p_d  = [dot_x_d; dot_y_d; dot_z_d];
% ddot_p_d = [ddot_x_d; ddot_y_d; ddot_z_d];

%% Lemniscata 2 (Experimento)

ampx = 0.5;
ampy = 1;
frecx = 2*pi/4;
frecy = 2*pi/8;
frecz = 2*pi/4;

x_d      = ampx*sin(frecx*t);
dot_x_d  = ampx*frecx*cos(frecx*t);
ddot_x_d = -ampx*frecx^2*sin(frecx*t);

y_d      = ampy*cos(frecy*t);
dot_y_d  = -ampy*frecy*sin(frecy*t);
ddot_y_d = -ampy*frecy^2*cos(frecy*t);

if (t>=0 && t<=5)
    z_d      = 1 - 0.7*exp(-0.1*t^3);
    dot_z_d  = 0.3*t^2*0.7*exp(-0.1*t^3);
    ddot_z_d = 0.3*0.7*(-0.1*3*exp(-0.1*t^3)*t^4 + 2*exp(-0.1*t^3)*t);
else
    z_d      = 1;
    dot_z_d  = 0;
    ddot_z_d = 0;
end

psi_d      = [0
              0
              0];
       
p_d      = [x_d; y_d; z_d];
dot_p_d  = [dot_x_d; dot_y_d; dot_z_d];
ddot_p_d = [ddot_x_d; ddot_y_d; ddot_z_d];

%% Disturbances
if (t>=60)
    delta_p = [sin(frecx*t)
               cos(frecy*t)
               sin(frecz*t)];

    d_eta = 0.045*sin(2.5*pi*t-3) + 0.09*sin(2*pi*t-7) + 0.135*sin(0.5*pi*t-9.5) + 0.09*sin(0.3*pi*t) + 0.054*sin(0.15*pi*t+4.5) + 0.045*sin(0.05*pi*t+2) + 0.135*sin(0.01*pi*t+3) + 0.225;
    delta_eta = [d_eta; d_eta; d_eta];
else
    delta_p = [0;0;0];
    delta_eta = [0;0;0];
end

== matlab function TwoLoopANNC_Integral_Paper/Subsystem/Adaptive RBFNN Control (Position) ==
  data: T output; p_d input; dot_p_d input; ddot_p_d input; tilde_p input; phi_d output; theta_d output; dot_hat_W output; dot_tilde_p input; eta input; hat_W input
function [T, phi_d,theta_d,dot_hat_W] = fcn(p_d, dot_p_d, ddot_p_d, tilde_p, dot_tilde_p, eta, hat_W)
m = 0.85*1.79;
g = 9.81;
%% RBFNN parameters
c      = [-1.5,-1,-0.5,0,0.5,1,1.5];
sigma  = 5*ones(length(c),1);
Lambda = diag([2.55 2.55 3.55]);
A      = 0.15;
Kv     = 1.257;
%%
phi   = eta(1);
theta = eta(2);
psi   = eta(3);

M  = diag([1/m 1/m cos(phi)*cos(theta)/m]);
e3 = [0;0;1];

Xin = [tilde_p' dot_tilde_p' p_d' dot_p_d' ddot_p_d'];
P = zeros(length(c),1);
for i=1:length(c)
    P(i) = exp(-(norm(Xin - c(i))^2)/sigma(i)^2);
end

gamma = dot_tilde_p + Lambda*tilde_p;

dot_hat_W = A*P*gamma';
hat_f = hat_W'*P;
u = M\(g*e3 + hat_f + Kv*gamma + ddot_p_d);

u1 = u(1)/u(3);
u2 = u(2)/u(3);

T = u(3);

phi_d   = asin(u1*sin(psi) - u2*cos(psi));
theta_d = asin((u1*cos(psi) + u2*sin(psi))/cos(phi_d));

== matlab function TwoLoopANNC_Integral_Paper/Subsystem/Integral SMC (Attitide) ==
  data: eta_d input; dot_eta_d input; tau output; eta input; dot_eta input; int_tilde_eta input; int_tilde_v input; dot_v_eta input; tilde_v output; v_eta output
function [tau, tilde_v, v_eta]  = fcn(eta_d, dot_eta_d, eta, dot_eta, int_tilde_eta, int_tilde_v, dot_v_eta)

Ixx = 0.03;
Iyy = Ixx;
Izz = 0.04;

kw    = 4.5;
kn    = 15;
rho_w = 0.000001;
rho_n = 0.0001;

phi   = eta(1);
theta = eta(2);

dot_phi   = dot_eta(1);
dot_theta = dot_eta(2);
dot_psi   = dot_eta(3);

M_eta = [Ixx 0 -Ixx*sin(theta);
         0 Iyy*cos(phi)^2+Izz*sin(phi)^2 (Iyy-Izz)*cos(phi)*sin(phi)*cos(theta);
         -Ixx*sin(theta) (Iyy-Izz)*cos(phi)*sin(phi)*cos(theta) Ixx*sin(theta)^2+Iyy*sin(phi)^2*cos(theta)^2+Izz*cos(phi)^2*cos(theta)^2];

C12 = (Iyy-Izz)*(dot_theta*cos(phi)*sin(phi)+dot_psi*sin(phi)^2*cos(theta))...
    + (Izz-Iyy)*dot_psi*cos(phi)^2*cos(theta)...
    - Ixx*dot_psi*cos(theta);

C13 = (Izz-Iyy)*dot_psi*cos(phi)*sin(phi)*cos(theta)^2;

C21 = (Izz-Iyy)*(dot_theta*cos(phi)*sin(phi)+dot_psi*sin(phi)^2*cos(theta))...
    + (Iyy-Izz)*dot_psi*cos(phi)^2*cos(theta)...
    + Ixx*dot_psi*cos(theta);

C22 = (Izz-Iyy)*dot_phi*cos(phi)*sin(phi);

C23 = -Ixx*dot_psi*sin(theta)*cos(theta)...
    + Iyy*dot_psi*sin(phi)^2*cos(theta)*sin(theta)...
    + Izz*dot_psi*cos(phi)^2*sin(theta)*cos(theta);

C31 = (Iyy-Izz)*dot_psi*cos(theta)^2*sin(phi)*cos(phi)...
    - Ixx*dot_theta*cos(theta);

C32 = (Izz-Iyy)*(dot_theta*cos(phi)*sin(phi)*sin(theta))...
    + (Iyy-Izz)*dot_phi*cos(phi)^2*cos(theta)...
    + Ixx*dot_psi*sin(theta)*cos(theta)...
    - Iyy*dot_psi*sin(phi)^2*sin(theta)*cos(theta)...
    - Izz*dot_theta*cos(phi)^2*sin(theta)*cos(theta);

C33 = (Iyy-Izz)*dot_phi*cos(phi)*sin(phi)*cos(theta)^2 ...
    - Iyy*dot_theta*sin(phi)^2*cos(theta)*sin(theta)...
    - Izz*dot_theta*cos(phi)^2*cos(theta)*sin(theta)...
    + Ixx*dot_theta*cos(theta)*sin(theta);

C_eta = [0   C12 C13;
         C21 C22 C23;
         C31 C32 C33];
     
tilde_eta = eta_d - eta;

s_w = tilde_eta + kw*int_tilde_eta;

v_eta = dot_eta_d + kw*tilde_eta + rho_w*sign(s_w);

tilde_v = v_eta - dot_eta;
     
s_n = tilde_v + kn*int_tilde_v;
     
tau = M_eta*dot_v_eta + C_eta*dot_eta + rho_n*sign(s_n) + kn*M_eta*tilde_v;
